simulink model "PID_Optimization_Model"  (R2024b)
settings: Solver=ode23t  StartTime=0.0  StopTime=10.0  MaxStep=0.001  RelTol=1e-3
libraries: fl_lib x7, nesl_utility x5, slpidlib x1
settings Model: Creator=Admin  LastModifiedBy=Admin
settings SolverCC: ZeroCrossAlgorithm=Adaptive
settings DebuggingCC: AlgebraicLoopMsg=none  IgnoredZcDiagnostic=none
settings SimscapeCC: ExplicitSolverDiagnosticOptions=none

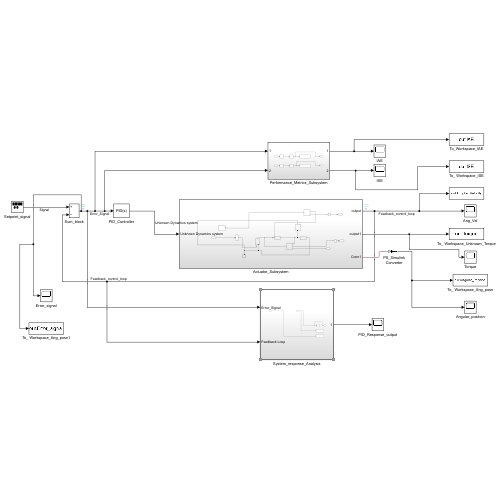
[thumbnail: Simulink's stored preview of the top-level diagram]
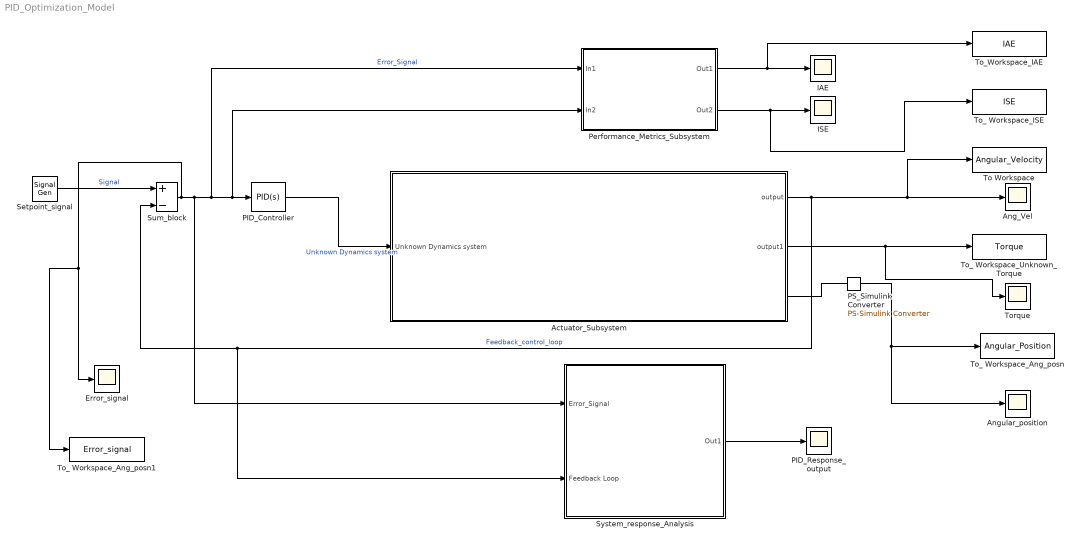
== system PID_Optimization_Model ==
  Actuator_Subsystem : Subsystem
  Ang_Vel : Scope
  Angular_position : Scope
  Error_signal : Scope
  IAE : Scope
  "ISE " : Scope
  PID_Controller : slpidlib/PID Controller  Controller=PID  Form=Parallel  TimeDomain=Continuous-time  UseExternalTs=off  SampleTime=-1  IntegratorMethod=Forward Euler  FilterMethod=Forward Euler  ControllerParametersSource=internal  P=100  I=100  UseKiTs=off  D=0  UseExternalDerivativeSource=off  N=100  UseFilter=on  TunerSelectOption=Transfer Function Based (PID Tuner App)  InitialConditionSource=internal  InitialConditionForIntegrator=0  InitialConditionForFilter=0  DifferentiatorICPrevScaledInput=0  ExternalReset=none  TrackingMode=off  Kt=1  LimitOutput=off  SatLimitsSource=internal  UpperSaturationLimit=inf  LowerSaturationLimit=-inf  LinearizeAsGain=on  AntiWindupMode=none  Kb=1  LimitIntegrator=off  UpperIntegratorSaturationLimit=inf  LowerIntegratorSaturationLimit=-inf  POutMin=[]  POutMax=[]  IOutMin=[]  IOutMax=[]  DOutMin=[]  DOutMax=[]  NOutMin=[]  NOutMax=[]  SumOutMin=[]  SumOutMax=[]  SaturationOutMin=[]  SaturationOutMax=[]  PParamMin=[]  PParamMax=[]  IParamMin=[]  IParamMax=[]  DParamMin=[]  DParamMax=[]  NParamMin=[]  NParamMax=[]  KbParamMin=[]  KbParamMax=[]  KtParamMin=[]  KtParamMax=[]  KbOutMin=[]  KbOutMax=[]  KtOutMin=[]  KtOutMax=[]  IntegratorOutMin=[]  IntegratorOutMax=[]  FilterOutMin=[]  FilterOutMax=[]  SumI1OutMin=[]  SumI1OutMax=[]  SumI2OutMin=[]  SumI2OutMax=[]  SumI3OutMin=[]  SumI3OutMax=[]  SumI4OutMin=[]  SumI4OutMax=[]  SumDOutMin=[]  SumDOutMax=[]  DifferentiatorOutMin=[]  DifferentiatorOutMax=[]  FilterDiffOutCoefMin=[]  FilterDiffOutCoefMax=[]  ReciprocalOutMin=[]  ReciprocalOutMax=[]  SumDenOutMin=[]  SumDenOutMax=[]  SumNumOutMin=[]  SumNumOutMax=[]  DivideOutMin=[]  DivideOutMax=[]  UdiffTsProdOutMin=[]  UdiffTsProdOutMax=[]  NTsProdOutMin=[]  NTsProdOutMax=[]  UintegralTsProdOutMin=[]  UintegralTsProdOutMax=[]  UngainTsProdOutMin=[]  UngainTsProdOutMax=[]  ClampingZeroOutDataTypeStr=Inherit: Inherit via back propagation  ClampingZeroOutMin=[]  ClampingZeroOutMax=[]  FilterDenConstantOutDataTypeStr=Inherit: Inherit via back propagation  FilterDenConstantOutMin=[]  FilterDenConstantOutMax=[]  PCopyOutDataTypeStr=Inherit: Inherit via back propagation  PCopyOutMin=[]  PCopyOutMax=[]  NCopyOutDataTypeStr=Inherit: Inherit via back propagation  NCopyOutMin=[]  NCopyOutMax=[]  IntegratorContinuousStateAttributes=''  IntegratorStateMustResolveToSignalObject=off  IntegratorRTWStateStorageClass=Auto  FilterContinuousStateAttributes=''  FilterStateMustResolveToSignalObject=off  FilterRTWStateStorageClass=Auto  ParallelPVariant=InternalParameters  IdealPVariant=Disabled  IVariant=InternalParameters  DVariant=InternalParameters  IntegratorVariant=Continuous  SatVariant=Disabled  AWVariant=Passthrough  PCopyVariant=Disabled  TRVariant=Disabled  FdbkBlocksVariant=Forward  IdealPFdbkVariant=Disabled  SatFdbkVariant=Disabled  DerivativeFilterVariant=ContFilter  NVariant=InternalParameters  NCopyVariant=Disabled  FilterICVariant=InternalICsFilter  IntegratorICVariant=InternalICs  ExternalResetVariant=Disabled  TRSumVariant=Passthrough  SumFdbkVariant=Disabled  SumVariant=Sum_PID  TsampFilterVariant=InternalTs  TsampNgainVariant=Passthrough  TsampIntegralVariant=Disabled_SignalSpec  ExternalSaturationOutDataTypeStr=Inherit: Same as second input  DerivativeSourceVariant=ErrorSignal  PreIntVariant=InternalPreInt
  PID_Response_output : Scope
  PS_Simulink Converter : nesl_utility/PS-Simulink Converter  PhysicalDomain=network_engine_domain  SubClassName=ps_output  LeftPortType=input  RightPortType=output  PseudoPeriodic=off  Frequencies=[]  VectorFormat=inherit  Unit=inherit  AffineConversion=off
  Performance_Metrics_Subsystem : Subsystem
  Setpoint_signal : SignalGenerator  WaveForm=sawtooth  Units=rad/sec
  Sum_block : Sum  Inputs=+-
  System_response_Analysis : Subsystem
  To Workspace : ToWorkspace  VariableName=Angular_Velocity  SaveFormat=Structure With Time  SampleTime=-1
  To_ Workspace_Ang_posn : ToWorkspace  VariableName=Angular_Position  SaveFormat=Structure With Time  SampleTime=-1
  To_ Workspace_Ang_posn1 : ToWorkspace  VariableName=Error_signal  SaveFormat=Structure With Time  SampleTime=-1
  To_ Workspace_ISE : ToWorkspace  VariableName=ISE  SaveFormat=Structure With Time  SampleTime=-1
  To_ Workspace_Unknown_Torque : ToWorkspace  VariableName=Torque  SaveFormat=Structure With Time  SampleTime=-1
  To_Workspace_IAE : ToWorkspace  VariableName=IAE  SaveFormat=Structure With Time  SampleTime=-1
  Torque : Scope
  wires:
  Sum_block/1 -> Performance_Metrics_Subsystem/1(In1), Performance_Metrics_Subsystem/2(In2), PID_Controller/1, System_response_Analysis/1(Error_Signal), To_ Workspace_Ang_posn1/1, Error_signal/1  "Error_Signal"
  Setpoint_signal/1 -> Sum_block/1  "Signal"
  Performance_Metrics_Subsystem/1(Out1) -> To_Workspace_IAE/1, IAE/1
  Performance_Metrics_Subsystem/2(Out2) -> To_ Workspace_ISE/1, "ISE "/1
  System_response_Analysis/1(Out1) -> PID_Response_output/1
  PID_Controller/1 -> Actuator_Subsystem/1(Unknown Dynamics system)  "Unknown Dynamics system"
  Actuator_Subsystem/1(output) -> System_response_Analysis/2(Feedback Loop), Sum_block/2, Ang_Vel/1, To Workspace/1  "Feedback_control_loop"
  PS_Simulink Converter/1 -> Angular_position/1, To_ Workspace_Ang_posn/1
  Actuator_Subsystem/2(output1) -> To_ Workspace_Unknown_Torque/1, Torque/1
  connections:
  PS_Simulink Converter/LConn1 -- Actuator_Subsystem/RConn1

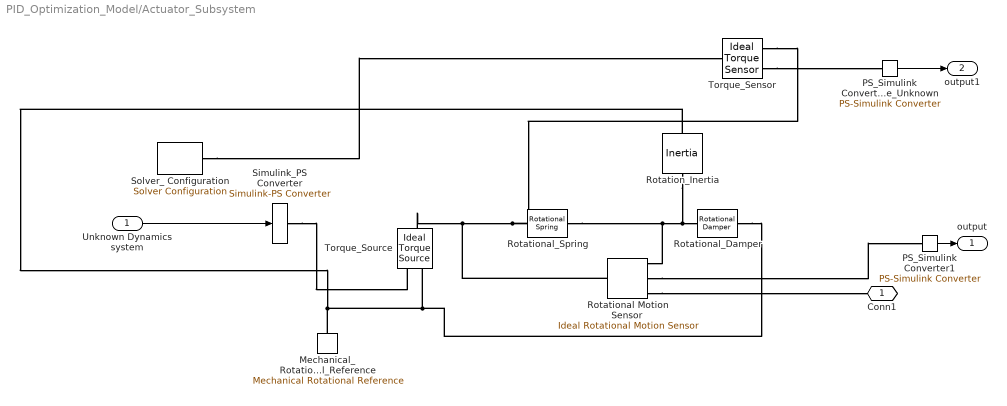
== system PID_Optimization_Model/Actuator_Subsystem ==
  Unknown Dynamics system : Inport
  Mechanical_ Rotational_Reference : fl_lib/Mechanical/Rotational Elements/Mechanical Rotational Reference
  PS_Simulink Converter1 : nesl_utility/PS-Simulink Converter  PhysicalDomain=network_engine_domain  SubClassName=ps_output  LeftPortType=input  RightPortType=output  PseudoPeriodic=off  Frequencies=[]  VectorFormat=inherit  Unit=inherit  AffineConversion=off
  PS_Simulink Converter_Torque_Unknown : nesl_utility/PS-Simulink Converter  PhysicalDomain=network_engine_domain  SubClassName=ps_output  LeftPortType=input  RightPortType=output  PseudoPeriodic=off  Frequencies=[]  VectorFormat=inherit  Unit=inherit  AffineConversion=off
  Rotation_Inertia : fl_lib/Mechanical/Rotational Elements/Inertia  inertia=0.01 kg*m^2  num_ports=foundation.enum.numPorts2.two  w_specify=on  w_priority=High  w=0 rad/s  w_nominal_specify=off  w_nominal_value=1  w_nominal_unit=rad/s  t_specify=off  t_priority=None  t=0 N*m  t_nominal_specify=off  t_nominal_value=1  t_nominal_unit=N*m
      settings: InternalSimscapePortConfiguration="{\"Bottom\":[],\"Left\":[{\"id\":\"I\",\"label\":\"\",\"type\":\"foundation.mechanical.rotational.rotational\"}],\"Right\":[{\"id\":\"J\",\"label\":\"\",\"type\":\"foundation.mechanical.rotational.rotational\"}],\"Top\":[]}"
  Rotational Motion Sensor : fl_lib/Mechanical/Mechanical Sensors/Ideal Rotational Motion Sensor  reference=foundation.enum.MeasurementReference.difference  acceleration_port=false  velocity_port=true  position_port=true  wrap_angle=true  offset=0 rad
  Rotational_Damper : fl_lib/Mechanical/Rotational Elements/Rotational Damper  D=0.001 N*m/(rad/s)  w_specify=on  w_priority=None  w=0 rad/s  w_nominal_specify=off  w_nominal_value=1  w_nominal_unit=rad/s  t_specify=off  t_priority=None  t=0 N*m  t_nominal_specify=off  t_nominal_value=1  t_nominal_unit=N*m
  Rotational_Spring : fl_lib/Mechanical/Rotational Elements/Rotational Spring  spr_rate=10 N*m/rad  w_specify=off  w_priority=None  w=0 rad/s  w_nominal_specify=off  w_nominal_value=1  w_nominal_unit=rad/s  t_specify=off  t_priority=None  t=0 N*m  t_nominal_specify=off  t_nominal_value=1  t_nominal_unit=N*m  phi_specify=off  phi_priority=High  phi=0 rad  phi_nominal_specify=off  phi_nominal_value=1  phi_nominal_unit=rad
  Simulink_PS Converter : nesl_utility/Simulink-PS Converter  PhysicalDomain=network_engine_domain  SubClassName=ps_input  LeftPortType=input  RightPortType=output  PseudoPeriodic=off  Frequencies=[]  NoiseDistribution=none  NoiseParameters=[]  Unit=N*m  AffineConversion=off  FilteringAndDerivatives=filter  SimscapeFilterOrder=2  InputFilterTimeConstant=0.001  UdotUserProvided=2
  Solver_ Configuration : nesl_utility/Solver Configuration  PhysicalDomain=network_engine_domain  SubClassName=solver  LeftPortType=input  RightPortType=generic  Tones=[]  Harmonics=[]  SimulateNoise=off  Profile=off  UseLocalSampling=off  EnableSwitchedLinearOptims=on  FrequencyDomain=off  UseCCode=off  RelTol=0.001  AbsTol=0.001  MinStep=1e-09  ToWorkspace=off  RevertToSquareIcSolve=off  NumHomotopyIterations=100  PhasorMode=off  PhasorModeNumHarmonics=1  ConsistencySolver=NEWTON_XTOL_AFTER_FTOL  IndexReductionMethod=DerivativeReplacement  DoDC=off  ResidualTolerance=1e-09  ConsistencyTolSource=GLOBAL  ConsistencyAbsTol=0.001  ConsistencyRelTol=0.001  ConsistencyTolFactor=0.001  UseLocalSolver=off  LocalSolverChoice=NE_BACKWARD_EULER_ADVANCER  ResolveIndetEquations=on  FunctionEvalNumThread=1  LocalSolverSampleTime=0.001  DoFixedCost=off  MaxNonlinIter=3  MaxModeIter=2  ComputeImpulses=off  ImpulseIterations=2  LinearAlgebra=auto  LinearAlgebraNumThread=0  EquationFormulation=NE_TIME_EF  DelaysMemoryBudget=1024  AutomaticFiltering=off  FilteringTimeConstant=0.001  PartitionStorageMethod=AS_NEEDED  PartitionMemoryBudget=1024  PartitionMethod=ROBUST  MultibodyUseLocalSolver=off  MultibodyLocalSolverChoice=ODE1  MultibodyLocalSolverSampleTime=0.001
  Torque_Sensor : fl_lib/Mechanical/Mechanical Sensors/Ideal Torque Sensor
  Torque_Source : fl_lib/Mechanical/Mechanical Sources/Ideal Torque Source
  Conn1 : PMIOPort  Side=Right
  output : Outport
  output1 : Outport  Port=2
  wires:
  Unknown Dynamics system/1 -> Simulink_PS Converter/1
  PS_Simulink Converter1/1 -> output/1
  PS_Simulink Converter_Torque_Unknown/1 -> output1/1
  connections:
  Mechanical_ Rotational_Reference/LConn1 -- Rotation_Inertia/LConn1 -- Rotational_Damper/RConn1 -- Torque_Source/RConn2
  Rotational Motion Sensor/RConn1 -- Rotation_Inertia/RConn1 -- Rotational_Damper/LConn1 -- Rotational_Spring/RConn1
  Rotational Motion Sensor/RConn2 -- PS_Simulink Converter1/LConn1
  Simulink_PS Converter/RConn1 -- Torque_Source/RConn1
  Rotational Motion Sensor/RConn3 -- Conn1/RConn1
  Torque_Source/LConn1 -- Torque_Sensor/RConn1 -- Rotational_Spring/LConn1 -- Rotational Motion Sensor/LConn1
  Torque_Sensor/RConn2 -- PS_Simulink Converter_Torque_Unknown/LConn1
  Solver_ Configuration/RConn1 -- Torque_Sensor/LConn1

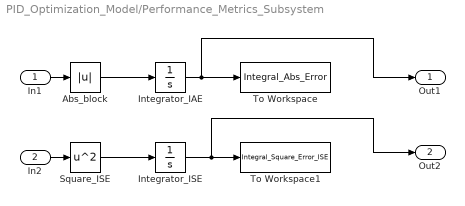
== system PID_Optimization_Model/Performance_Metrics_Subsystem ==
  In1 : Inport
  In2 : Inport  Port=2
  Abs_block : Abs  SaturateOnIntegerOverflow=off
  Integrator_IAE : Integrator
  Integrator_ISE : Integrator
  Square_ISE : Math  Operator=square
  To Workspace : ToWorkspace  VariableName=Integral_Abs_Error  SaveFormat=Timeseries  SampleTime=-1
  To Workspace1 : ToWorkspace  VariableName=Integral_Square_Error_ISE  SaveFormat=Timeseries  SampleTime=-1
  Out1 : Outport
  Out2 : Outport  Port=2
  wires:
  Abs_block/1 -> Integrator_IAE/1
  Integrator_IAE/1 -> Out1/1, To Workspace/1
  In1/1 -> Abs_block/1
  Square_ISE/1 -> Integrator_ISE/1
  Integrator_ISE/1 -> Out2/1, To Workspace1/1
  In2/1 -> Square_ISE/1

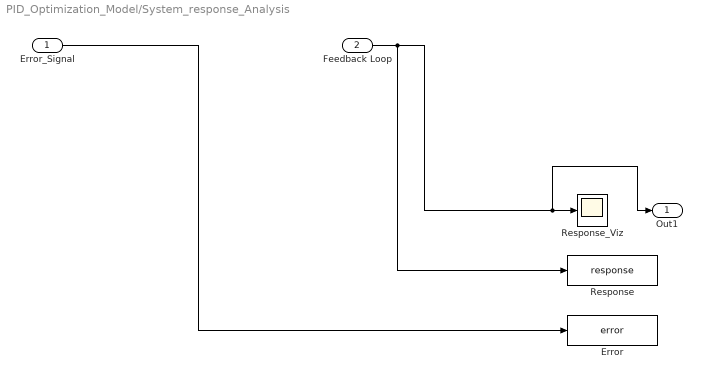
== system PID_Optimization_Model/System_response_Analysis ==
  Error_Signal : Inport
  Feedback Loop : Inport  Port=2
  Error : ToWorkspace  VariableName=error  SaveFormat=Timeseries  SampleTime=-1
  Response : ToWorkspace  VariableName=response  SaveFormat=Timeseries  SampleTime=-1
  Response_Viz : Scope
  Out1 : Outport
  wires:
  Feedback Loop/1 -> Response/1, Out1/1, Response_Viz/1
  Error_Signal/1 -> Error/1
